simulink model "model63"  (R2016a)
settings: Solver=VariableStepAuto  StartTime=0.0  StopTime=900.0  RelTol=1e-3
values from neighbouring files (symbols this model uses):
  m0 = 408600    [opt63_run.m]
  m0_inv = 1/m0    (= 2.44738130201e-06)    [opt63_run.m]
undefined symbols (not defined in the file or in its folder): h_array, h_g, h_rho
libraries: aerolibatmos2 x1
settings Model: Creator=normal  LastModifiedBy=normal

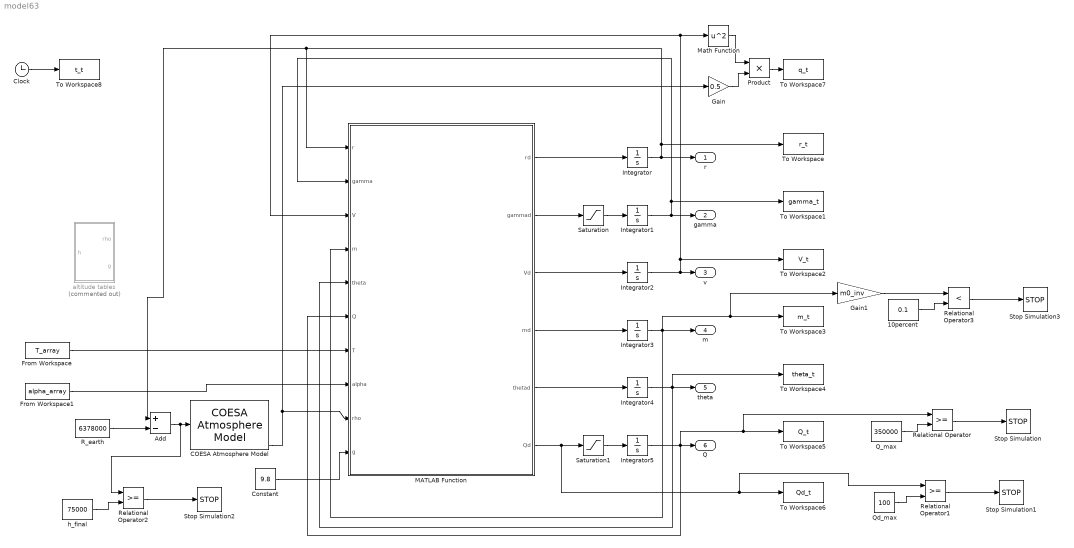
== system model63 ==
  10percent : Constant  Value=0.1
  Add : Sum  Inputs=+-
  COESA Atmosphere Model : aerolibatmos2/COESA Atmosphere Model  units=Metric (MKS)  spec=1976 COESA-extended U.S. Standard Atmosphere  model=Profile  profile_var=High temperature  profile_percent=1%  profile_alt=5 km (16404 ft)  envelope_var=High temperature  envelope_percent=1%  action=Warning
  Clock : Clock
  Constant : Constant  Value=9.8
  From Workspace : FromWorkspace  VariableName=T_array  SampleTime=0
  From Workspace1 : FromWorkspace  VariableName=alpha_array  SampleTime=0
  Gain : Gain  Gain=0.5
  Gain1 : Gain  Gain=m0_inv
  Integrator : Integrator  InitialCondition=6398000
  Integrator1 : Integrator  InitialCondition=0.088
  Integrator2 : Integrator  InitialCondition=1475.5
  Integrator3 : Integrator  InitialCondition=m0
  Integrator4 : Integrator
  Integrator5 : Integrator
  MATLAB Function : MATLAB Function  TreatAsAtomicUnit=on
  Math Function : Math  Operator=square  SaturateOnIntegerOverflow=on
  Product : Product
  Q_max : Constant  Value=350000
  Qd_max : Constant  Value=100
  R_earth : Constant  Value=6378000
  Relational Operator : RelationalOperator  OutDataTypeStr=boolean
  Relational Operator1 : RelationalOperator  OutDataTypeStr=boolean
  Relational Operator2 : RelationalOperator  OutDataTypeStr=boolean
  Relational Operator3 : RelationalOperator  Operator=<  OutDataTypeStr=boolean
  Saturation : Saturate  UpperLimit=0.05  LowerLimit=-0.05
  Saturation1 : Saturate  UpperLimit=5000  LowerLimit=0
  Stop Simulation{,1..3} (4 alike) : Stop
  To Workspace : ToWorkspace  VariableName=r_t  SampleTime=-1
  To Workspace1 : ToWorkspace  VariableName=gamma_t  SampleTime=-1
  To Workspace2 : ToWorkspace  VariableName=V_t  SampleTime=-1
  To Workspace3 : ToWorkspace  VariableName=m_t  SampleTime=-1
  To Workspace4 : ToWorkspace  VariableName=theta_t  SampleTime=-1
  To Workspace5 : ToWorkspace  VariableName=Q_t  SampleTime=-1
  To Workspace6 : ToWorkspace  VariableName=Qd_t  SampleTime=-1
  To Workspace7 : ToWorkspace  VariableName=q_t  SampleTime=-1
  To Workspace8 : ToWorkspace  VariableName=t_t  SampleTime=-1
  altitude tables : Subsystem  Commented=on
  h_final : Constant  Value=75000
  r : Outport
  gamma : Outport  Port=2
  v : Outport  Port=3
  m : Outport  Port=4
  theta : Outport  Port=5
  Q : Outport  Port=6
  wires:
  Integrator/1 -> MATLAB Function/1(r), Add/1, To Workspace/1, r/1
  Integrator1/1 -> MATLAB Function/2(gamma), To Workspace1/1, gamma/1
  Integrator2/1 -> Math Function/1, MATLAB Function/3(V), To Workspace2/1, v/1
  Integrator4/1 -> MATLAB Function/5(theta), To Workspace4/1, theta/1
  MATLAB Function/5(thetad) -> Integrator4/1
  From Workspace/1 -> MATLAB Function/7(T)
  From Workspace1/1 -> MATLAB Function/8(alpha)
  COESA Atmosphere Model/4 -> Gain/1, MATLAB Function/9(rho)
  Constant/1 -> MATLAB Function/10(g)
  MATLAB Function/1(rd) -> Integrator/1
  MATLAB Function/2(gammad) -> Saturation/1
  MATLAB Function/3(Vd) -> Integrator2/1
  MATLAB Function/4(md) -> Integrator3/1
  Add/1 -> COESA Atmosphere Model/1, Relational Operator2/1
  R_earth/1 -> Add/2
  Product/1 -> To Workspace7/1
  Gain/1 -> Product/2
  Math Function/1 -> Product/1
  Clock/1 -> To Workspace8/1
  Integrator5/1 -> MATLAB Function/6(Q), Relational Operator/1, To Workspace5/1, Q/1
  Relational Operator/1 -> Stop Simulation/1
  Q_max/1 -> Relational Operator/2
  MATLAB Function/6(Qd) -> Relational Operator1/1, To Workspace6/1, Saturation1/1
  Relational Operator1/1 -> Stop Simulation1/1
  Qd_max/1 -> Relational Operator1/2
  Relational Operator2/1 -> Stop Simulation2/1
  h_final/1 -> Relational Operator2/2
  Saturation/1 -> Integrator1/1
  Saturation1/1 -> Integrator5/1
  Integrator3/1 -> MATLAB Function/4(m), Gain1/1, To Workspace3/1, m/1
  Relational Operator3/1 -> Stop Simulation3/1
  10percent/1 -> Relational Operator3/2
  Gain1/1 -> Relational Operator3/1

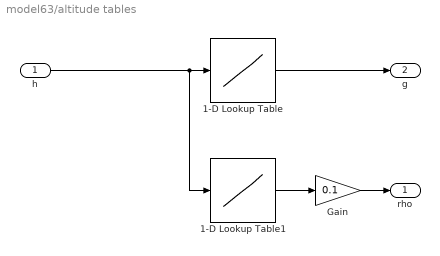
== system model63/altitude tables ==
  h : Inport
  1-D Lookup Table : Lookup_n-D  NumberOfTableDimensions=1  BreakpointsForDimension1=h_array  Table=h_g(h_array)  InternalRulePriority=Speed  RndMeth=Simplest  InputSameDT=on
  1-D Lookup Table1 : Lookup_n-D  NumberOfTableDimensions=1  BreakpointsForDimension1=h_array  Table=h_rho(h_array)  InternalRulePriority=Speed  RndMeth=Simplest  InputSameDT=on
  Gain : Gain  Gain=0.1
  rho : Outport
  g : Outport  Port=2
  wires:
  h/1 -> 1-D Lookup Table1/1, 1-D Lookup Table/1
  1-D Lookup Table/1 -> g/1
  1-D Lookup Table1/1 -> Gain/1
  Gain/1 -> rho/1

== matlab function model63/MATLAB Function ==
  data: r input; gamma input; V input; m input; theta input; Q input; rd output; T input; alpha input; rho input; g input; gammad output; Vd output; md output; thetad output; Qd output
function [rd,gammad,Vd,md,thetad,Qd] = model_states(r,gamma,V,m,theta,Q,T,alpha,rho,g)
Isp=450;
Cq=5.79e-8; %take care of units
g0=9.81; %check
S=860;

Cl=-0.0041065+0.933*alpha+0.854*alpha^2;
Cd=0.080505-0.03026*Cl+0.086495*Cl^2;
qs=0.5*rho*V^2;
D=qs*Cd*S;
L=qs*Cl*S;

rd=V*sin(gamma);
gammad=L/(m*V)+(V/r-g/V)*cos(gamma);
Vd=(T-D)/m-g*sin(gamma);
md=-T/(Isp*g0);
thetad=(V*cos(gamma))/r;
Qd=Cq*sqrt(abs(rho))*V^3;

end
